simulink model "TD3"  (R2017b)
settings: Solver=VariableStepAuto  StartTime=0.0  StopTime=10.0  RelTol=1e-3
undefined symbols (not defined in the file): Cr, J, p, phi, PI
settings Model: Creator=TP-EO-5  LastModifiedBy=TP-EO-5

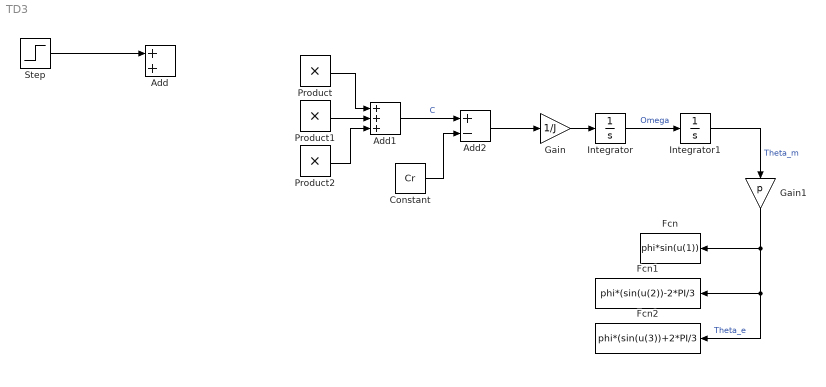
== system TD3 ==
  Add : Sum
  Add1 : Sum  Inputs=+++
  Add2 : Sum  Inputs=+-
  Constant : Constant  Value=Cr
  Fcn : Fcn  Expr=phi*sin(u(1))
  Fcn1 : Fcn  Expr=phi*(sin(u(2))-2*PI/3
  Fcn2 : Fcn  Expr=phi*(sin(u(3))+2*PI/3
  Gain : Gain  Gain=1/J
  Gain1 : Gain  Gain=p
  Integrator : Integrator
  Integrator1 : Integrator
  Product : Product
  Product1 : Product
  Product2 : Product
  Step : Step  SampleTime=0
  wires:
  Step/1 -> Add/1
  Product/1 -> Add1/1
  Add1/1 -> Add2/1  "C"
  Add2/1 -> Gain/1
  Gain/1 -> Integrator/1
  Integrator/1 -> Integrator1/1  "Omega"
  Constant/1 -> Add2/2
  Product1/1 -> Add1/2
  Product2/1 -> Add1/3
  Integrator1/1 -> Gain1/1  "Theta_m"
  Gain1/1 -> Fcn2/1, Fcn1/1, Fcn/1  "Theta_e"
